simulink model "FIXEDPOINT_THIRD_ORDER_SIGMADELTA"  (R2021b)
settings: Solver=VariableStepAuto  StartTime=0.0  StopTime=0.1  MaxStep=1e-8  RelTol=1e-3
libraries: fl_lib x9, nesl_utility x4, simulink x1
settings Model: FPTShortcutValueString='{{},{''BaselineRun'',1,1,1,''BaselineRun'','''',{},''M'','''',''''},{''EmbeddedRun'',1,1,1,''EmbeddedRun'','''',{},''M'','''',''''}}'  Creator=caccolillo  LastModifiedBy=caccolillo
settings OptimizationCC: BlockReduction=off  ConditionallyExecuteInputs=off
settings DebuggingCC: SignalRangeChecking=warning

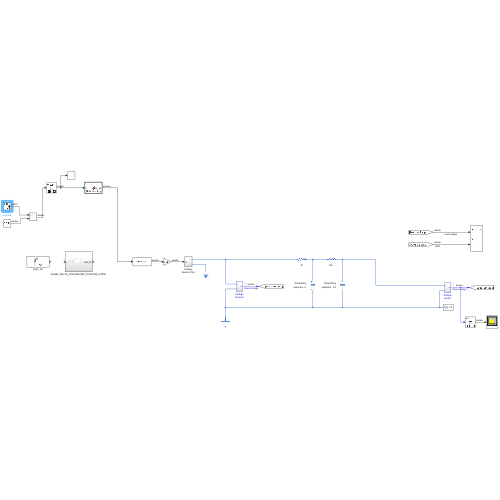
[thumbnail: Simulink's stored preview of the top-level diagram]
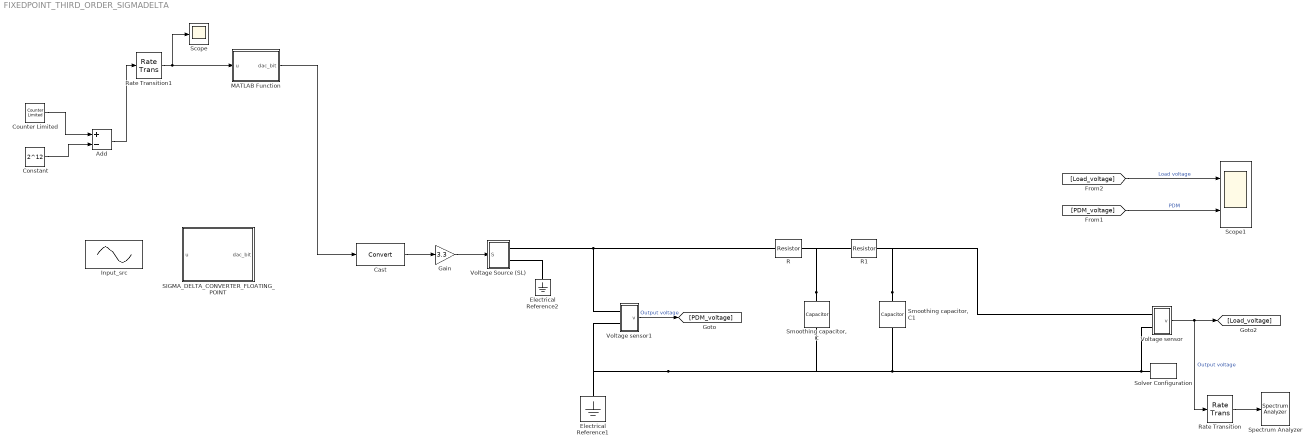
== system FIXEDPOINT_THIRD_ORDER_SIGMADELTA ==
  Add : Sum  Inputs=+-
  Cast : DataTypeConversion
  Constant : Constant  Value=2^12
  Counter Limited : simulink/Sources/Counter Limited  uplimit=2^13  tsamp=1/32000
  Electrical Reference1 : fl_lib/Electrical/Electrical Elements/Electrical Reference
  Electrical Reference2 : fl_lib/Electrical/Electrical Elements/Electrical Reference
  Gain : Gain  Gain=3.3
  Input_src : Sin  Amplitude=1024  Frequency=2*pi*1000  SampleTime=2e-07
  MATLAB Function : MATLAB Function  TreatAsAtomicUnit=on
  R : fl_lib/Electrical/Electrical Elements/Resistor  R=1 kOhm  i_specify=off  i_priority=High  i=0 A  i_nominal_specify=off  i_nominal_unit=A  i_nominal_value=1  v_specify=off  v_priority=High  v=0 V  v_nominal_specify=off  v_nominal_unit=V  v_nominal_value=1
  R1 : fl_lib/Electrical/Electrical Elements/Resistor  R=1 kOhm  i_specify=off  i_priority=High  i=0 A  i_nominal_specify=off  i_nominal_unit=A  i_nominal_value=1  v_specify=off  v_priority=High  v=0 V  v_nominal_specify=off  v_nominal_unit=V  v_nominal_value=1
  Rate Transition : RateTransition  Deterministic=off  OutPortSampleTime=1/100e3
  Rate Transition1 : RateTransition  Deterministic=off
  SIGMA_DELTA_CONVERTER_FLOATING_POINT : Subsystem
  Scope : Scope
  Scope1 : Scope  NumInputPorts=2
  "Smoothing capacitor, C" : fl_lib/Electrical/Electrical Elements/Capacitor  c=10 nF  r=0 Ohm  g=0 1/Ohm  i_specify=off  i_priority=High  i=0 A  i_nominal_specify=off  i_nominal_unit=A  i_nominal_value=1  v_specify=off  v_priority=High  v=0 V  v_nominal_specify=off  v_nominal_unit=V  v_nominal_value=1  vc_specify=on  vc_priority=High  vc=0 V  vc_nominal_specify=off  vc_nominal_unit=V  vc_nominal_value=1
  "Smoothing capacitor, C1" : fl_lib/Electrical/Electrical Elements/Capacitor  c=10 nF  r=0 Ohm  g=0 1/Ohm  i_specify=off  i_priority=High  i=0 A  i_nominal_specify=off  i_nominal_unit=A  i_nominal_value=1  v_specify=off  v_priority=High  v=0 V  v_nominal_specify=off  v_nominal_unit=V  v_nominal_value=1  vc_specify=on  vc_priority=High  vc=0 V  vc_nominal_specify=off  vc_nominal_unit=V  vc_nominal_value=1
  Solver Configuration : nesl_utility/Solver Configuration  PhysicalDomain=network_engine_domain  SubClassName=solver  LeftPortType=input  RightPortType=generic  Tones=[]  Harmonics=[]  SimulateNoise=off  Profile=off  UseLocalSampling=off  EnableSwitchedLinearOptims=on  FrequencyDomain=off  UseCCode=off  RelTol=0.001  AbsTol=1e-06  MinStep=1e-09  ToWorkspace=off  RevertToSquareIcSolve=off  NumHomotopyIterations=100  PhasorMode=off  PhasorModeNumHarmonics=1  DoDC=off  ResidualTolerance=1e-9  UseLocalSolver=off  LocalSolverChoice=NE_BACKWARD_EULER_ADVANCER  LocalSolverSampleTime=1e-7  DoFixedCost=off  MaxNonlinIter=12  MaxModeIter=2  ComputeImpulses=off  ImpulseIterations=2  LinearAlgebra=Sparse  EquationFormulation=NE_TIME_EF  DelaysMemoryBudget=1024  AutomaticFiltering=on  FilteringTimeConstant=0.001  PartitionStorageMethod=AS_NEEDED  PartitionMemoryBudget=1024  PartitionMethod=FAST
      settings: SourceProductBaseCode=PW,SS
  Spectrum Analyzer : SpectrumAnalyzer
  Voltage Source (SL) : Subsystem
      settings: CopyFcn=set_param(gcb,'LinkStatus','none')
  Voltage sensor : Subsystem
      settings: CopyFcn=set_param(gcb,'LinkStatus','none')
  Voltage sensor1 : Subsystem
      settings: CopyFcn=set_param(gcb,'LinkStatus','none')
  wires:
  [PDM_voltage] -> Scope1/2  "PDM"
  Rate Transition/1 -> Spectrum Analyzer/1
  Voltage sensor/1(v) -> Rate Transition/1, [Load_voltage]  "Output voltage"
  Voltage sensor1/1(v) -> [PDM_voltage]  "Output voltage"
  Gain/1 -> Voltage Source (SL)/1(S)
  [Load_voltage] -> Scope1/1  "Load voltage"
  Cast/1 -> Gain/1
  Add/1 -> Rate Transition1/1
  MATLAB Function/1(dac_bit) -> Cast/1
  Counter Limited/1 -> Add/1
  Constant/1 -> Add/2
  Rate Transition1/1 -> Scope/1, MATLAB Function/1(u)
  connections:
  Solver Configuration/RConn1 -- Voltage sensor1/LConn2 -- Electrical Reference1/LConn1 -- "Smoothing capacitor, C"/RConn1 -- "Smoothing capacitor, C1"/RConn1 -- Voltage sensor/LConn2
  "Smoothing capacitor, C"/LConn1 -- R/LConn1 -- R1/RConn1
  "Smoothing capacitor, C1"/LConn1 -- R1/LConn1 -- Voltage sensor/LConn1
  Voltage sensor1/LConn1 -- R/RConn1 -- Voltage Source (SL)/RConn1
  Voltage Source (SL)/RConn2 -- Electrical Reference2/LConn1

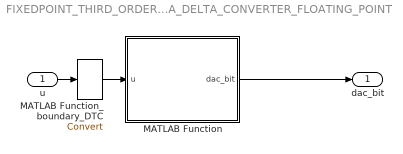
== system FIXEDPOINT_THIRD_ORDER_SIGMADELTA/SIGMA_DELTA_CONVERTER_FLOATING_POINT ==
  u : Inport
  MATLAB Function : Subsystem  TreatAsAtomicUnit=on  Variant=on  VariantControlMode=label  VariantControl=Choice  LabelModeActiveChoice=(default)
  MATLAB Function_boundary_DTC : DataTypeConversion  SaturateOnIntegerOverflow=on  RndMeth=Zero
  dac_bit : Outport
  wires:
  u/1 -> MATLAB Function_boundary_DTC/1
  MATLAB Function_boundary_DTC/1 -> MATLAB Function/1(u)
  MATLAB Function/1(dac_bit) -> dac_bit/1

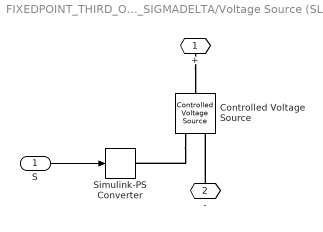
== system FIXEDPOINT_THIRD_ORDER_SIGMADELTA/Voltage Source (SL) ==
  S : Inport
  Controlled Voltage Source : fl_lib/Electrical/Electrical Sources/Controlled Voltage Source
  Simulink-PS Converter : nesl_utility/Simulink-PS Converter  PhysicalDomain=network_engine_domain  SubClassName=ps_input  LeftPortType=input  RightPortType=output  PseudoPeriodic=off  Frequencies=[]  NoiseDistribution=none  NoiseParameters=[]  Unit=V  AffineConversion=off  FilteringAndDerivatives=zero  SimscapeFilterOrder=1  InputFilterTimeConstant=.001  UdotUserProvided=0
      settings: SourceProductBaseCode=PW,SS
  + : PMIOPort  Side=Right
  - : PMIOPort  Port=2  Side=Right
  wires:
  S/1 -> Simulink-PS Converter/1
  connections:
  +/RConn1 -- Controlled Voltage Source/LConn1
  -/RConn1 -- Controlled Voltage Source/RConn2
  Controlled Voltage Source/RConn1 -- Simulink-PS Converter/RConn1

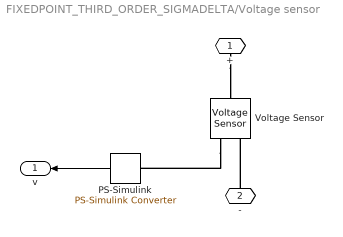
== system FIXEDPOINT_THIRD_ORDER_SIGMADELTA/Voltage sensor ==
  PS-Simulink : nesl_utility/PS-Simulink Converter  PhysicalDomain=network_engine_domain  SubClassName=ps_output  LeftPortType=input  RightPortType=output  PseudoPeriodic=off  Frequencies=[]  Unit=V  AffineConversion=off
      settings: SourceProductBaseCode=PW,SS
  Voltage Sensor : fl_lib/Electrical/Electrical Sensors/Voltage Sensor
  + : PMIOPort  Side=Left
  - : PMIOPort  Port=2  Side=Left
  v : Outport
  wires:
  PS-Simulink/1 -> v/1
  connections:
  Voltage Sensor/RConn1 -- PS-Simulink/LConn1
  +/RConn1 -- Voltage Sensor/LConn1
  -/RConn1 -- Voltage Sensor/RConn2

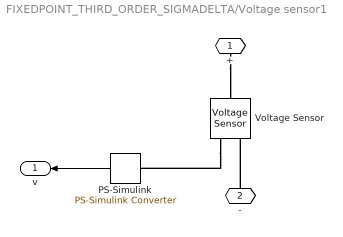
== system FIXEDPOINT_THIRD_ORDER_SIGMADELTA/Voltage sensor1 ==
  PS-Simulink : nesl_utility/PS-Simulink Converter  PhysicalDomain=network_engine_domain  SubClassName=ps_output  LeftPortType=input  RightPortType=output  PseudoPeriodic=off  Frequencies=[]  Unit=V  AffineConversion=off
      settings: SourceProductBaseCode=PW,SS
  Voltage Sensor : fl_lib/Electrical/Electrical Sensors/Voltage Sensor
  + : PMIOPort  Side=Left
  - : PMIOPort  Port=2  Side=Left
  v : Outport
  wires:
  PS-Simulink/1 -> v/1
  connections:
  Voltage Sensor/RConn1 -- PS-Simulink/LConn1
  +/RConn1 -- Voltage Sensor/LConn1
  -/RConn1 -- Voltage Sensor/RConn2

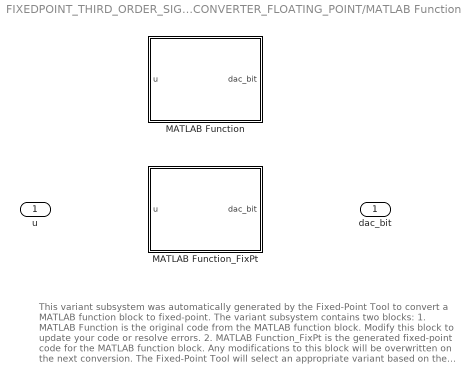
== system FIXEDPOINT_THIRD_ORDER_SIGMADELTA/SIGMA_DELTA_CONVERTER_FLOATING_POINT/MATLAB Function ==
  note: This variant subsystem was automatically generated by the Fixed-Point Tool to convert a MATLAB function block to fixed-point.
      |
      | The variant subsystem contains two blocks:
      | 1. MATLAB Function is the original code from the MATLAB function block. Modify this block to update your code or resolve errors.
      |
      | 2. MATLAB Function_FixPt is the generated fixed-point code for the MATLAB function block. Any modifications to this block will be overwritten on the next conversion.
      |
      | The Fixed-Point Tool will select an appropriate variant based on the Model Settings. Learn more. .
  u : Inport
  MATLAB Function : MATLAB Function  TreatAsAtomicUnit=on  VariantControl=false()
  MATLAB Function_FixPt : MATLAB Function  TreatAsAtomicUnit=on  VariantControl=(default)
  dac_bit : Outport

== matlab function FIXEDPOINT_THIRD_ORDER_SIGMADELTA/SIGMA_DELTA_CONVERTER_FLOATING_POINT/MATLAB Function/MATLAB Function_FixPt ==
  settings: fimath=fimath('RoundingMethod', 'Floor', 'OverflowAction', 'Wrap', 'ProductMode', 'FullPrecision', 'MaxProductWordLength', 128, 'SumMode', 'FullPrecision', 'MaxSumWordLength', 128)
  data: u input; dac_bit output
%auto-generated
function dac_bit = SDM_fcn_fixpt(u)  %#codegen
% Auto-generated by DESIGN_THIRD_ORDER.m
% 3rd-order CIFB sigma-delta modulator - FLOATING POINT REFERENCE
%
% This file is the floating-point golden model intended for use with
% MATLAB Fixed-Point Designer ("Convert to Fixed Point" workflow).
% All arithmetic uses double precision so the tool can instrument the
% function, observe min/max ranges, and propose data types.
%
% Input  u : signed integer count from the 13-bit ADC,
%            range [-4096, 4095]. Internally normalised to [-1,+1).
% Output : single bit (logical) for 1-bit DAC drive.
%
% Suggested starting types for Fixed-Point Designer:
%   u           : fixdt(1, 13, 0)
%   coefficients: fixdt(1, 18, 14)
%   int1..int3  : fixdt(1, 32, 14)

fm = get_fimath();
u = fi(u, 1, 16, 4, fm);

dac_bit = false;

persistent int1 int2 int3
if isempty(int1)
    int1 = fi(0, 1, 16, 15, fm);
    int2 = fi(0, 1, 16, 16, fm);
    int3 = fi(0, 1, 16, 17, fm);
end

% Floating-point coefficients (scaled CIFB, 3rd order)
B1 = fi(0.172222623529955, 0, 16, 18, fm);
A1 = fi(0.172222623529955, 0, 16, 18, fm);
A2 = fi(0.123562088507108, 0, 16, 18, fm);
A3 = fi(0.122457379474687, 0, 16, 19, fm);
C1 = fi(0.10952288682635, 0, 16, 19, fm);
C2 = fi(0.357050181625205, 0, 16, 17, fm);
G1 = fi(4.2457997600222e-05, 0, 16, 30, fm);

% Saturate and normalise the 13-bit signed input to [-1, +1)
u_sat = fi(max(min(double(u), fi(4095, 0, 12, 0, fm)), fi(-4096, 1, 13, 0, fm)), 1, 16, 4, fm);
u_norm = fi(fi_div_by_shift(u_sat, 12), 1, 16, 16, fm);

% Quantizer decision based on the last integrator (int3)
if int3 >= fi(0, 0, 1, 0, fm)
    dac_bit(:) = true;
    v       =  fi(1, 1, 16, 14, fm);
else
    dac_bit(:) = false;
    v       = fi(-1, 1, 16, 14, fm);
end

% Integrator 1: int1 += B1*u - A1*v
int1(:) = fi_signed(int1 + B1*u_norm) - A1*v;

% Integrator 2: int2 += C1*int1 - A2*v
int2(:) = fi_signed(int2 + C1*int1) - A2*v;

% Integrator 3: int3 += C2*int2 - G1*int3 - A3*v
% G1 is the resonator local feedback that places NTF zeros
% at non-DC frequencies inside the signal band.
int3(:) = fi_signed(fi_signed(int3 + C2*int2) - G1*int3) - A3*v;

end



function y = fi_div_by_shift(a,shift_len)
    coder.inline( 'always' );
    if isfi( a )
        nt = numerictype( a );
        fm = fimath( a );
        nt_bs = numerictype( nt.Signed, nt.WordLength + shift_len, nt.FractionLength + shift_len );
        y = bitsra( fi( a, nt_bs, fm ), shift_len );
    else
        y = a / 2 ^ shift_len;
    end
end


function y = fi_signed(a)
    coder.inline( 'always' );
    if isfi( a ) && ~(issigned( a ))
        nt = numerictype( a );
        new_nt = numerictype( 1, nt.WordLength + 1, nt.FractionLength );
        y = fi( a, new_nt, fimath( a ) );
    else
        y = a;
    end
end

function fm = get_fimath()
	fm = fimath('RoundingMethod', 'Floor',...
	     'OverflowAction', 'Wrap',...
	     'ProductMode','FullPrecision',...
	     'MaxProductWordLength', 128,...
	     'SumMode','FullPrecision',...
	     'MaxSumWordLength', 128);
end

== matlab function FIXEDPOINT_THIRD_ORDER_SIGMADELTA/MATLAB Function ==
  data: u input; dac_bit output
%auto-generated
function dac_bit = SDM_fcn_fixpt(u)  %#codegen
% Auto-generated by DESIGN_THIRD_ORDER.m
% 3rd-order CIFB sigma-delta modulator - FLOATING POINT REFERENCE
%
% This file is the floating-point golden model intended for use with
% MATLAB Fixed-Point Designer ("Convert to Fixed Point" workflow).
% All arithmetic uses double precision so the tool can instrument the
% function, observe min/max ranges, and propose data types.
%
% Input  u : signed integer count from the 13-bit ADC,
%            range [-4096, 4095]. Internally normalised to [-1,+1).
% Output : single bit (logical) for 1-bit DAC drive.
%
% Suggested starting types for Fixed-Point Designer:
%   u           : fixdt(1, 13, 0)
%   coefficients: fixdt(1, 18, 14)
%   int1..int3  : fixdt(1, 32, 14)

fm = get_fimath();
u = fi(u, 1, 16, 4, fm);

dac_bit = false;

persistent int1 int2 int3
if isempty(int1)
    int1 = fi(0, 1, 16, 15, fm);
    int2 = fi(0, 1, 16, 16, fm);
    int3 = fi(0, 1, 16, 17, fm);
end

% Floating-point coefficients (scaled CIFB, 3rd order)
B1 = fi(0.172222623529955, 0, 16, 18, fm);
A1 = fi(0.172222623529955, 0, 16, 18, fm);
A2 = fi(0.123562088507108, 0, 16, 18, fm);
A3 = fi(0.122457379474687, 0, 16, 19, fm);
C1 = fi(0.10952288682635, 0, 16, 19, fm);
C2 = fi(0.357050181625205, 0, 16, 17, fm);
G1 = fi(4.2457997600222e-05, 0, 16, 30, fm);

% Saturate and normalise the 13-bit signed input to [-1, +1)
u_sat = fi(max(min(double(u), fi(4095, 0, 12, 0, fm)), fi(-4096, 1, 13, 0, fm)), 1, 16, 4, fm);
u_norm = fi(fi_div_by_shift(u_sat, 12), 1, 16, 16, fm);

% Quantizer decision based on the last integrator (int3)
if int3 >= fi(0, 0, 1, 0, fm)
    dac_bit(:) = true;
    v       =  fi(1, 1, 16, 14, fm);
else
    dac_bit(:) = false;
    v       = fi(-1, 1, 16, 14, fm);
end

% Integrator 1: int1 += B1*u - A1*v
int1(:) = fi_signed(int1 + B1*u_norm) - A1*v;

% Integrator 2: int2 += C1*int1 - A2*v
int2(:) = fi_signed(int2 + C1*int1) - A2*v;

% Integrator 3: int3 += C2*int2 - G1*int3 - A3*v
% G1 is the resonator local feedback that places NTF zeros
% at non-DC frequencies inside the signal band.
int3(:) = fi_signed(fi_signed(int3 + C2*int2) - G1*int3) - A3*v;

end



function y = fi_div_by_shift(a,shift_len)
    coder.inline( 'always' );
    if isfi( a )
        nt = numerictype( a );
        fm = fimath( a );
        nt_bs = numerictype( nt.Signed, nt.WordLength + shift_len, nt.FractionLength + shift_len );
        y = bitsra( fi( a, nt_bs, fm ), shift_len );
    else
        y = a / 2 ^ shift_len;
    end
end


function y = fi_signed(a)
    coder.inline( 'always' );
    if isfi( a ) && ~(issigned( a ))
        nt = numerictype( a );
        new_nt = numerictype( 1, nt.WordLength + 1, nt.FractionLength );
        y = fi( a, new_nt, fimath( a ) );
    else
        y = a;
    end
end

function fm = get_fimath()
	fm = fimath('RoundingMethod', 'Floor',...
	     'OverflowAction', 'Wrap',...
	     'ProductMode','FullPrecision',...
	     'MaxProductWordLength', 128,...
	     'SumMode','FullPrecision',...
	     'MaxSumWordLength', 128);
end

== matlab function FIXEDPOINT_THIRD_ORDER_SIGMADELTA/SIGMA_DELTA_CONVERTER_FLOATING_POINT/MATLAB Function/MATLAB Function ==
  data: u input; dac_bit output
function dac_bit = SDM_fcn(u)  %#codegen
% Auto-generated by DESIGN_THIRD_ORDER.m
% 3rd-order CIFB sigma-delta modulator - FLOATING POINT REFERENCE
%
% This file is the floating-point golden model intended for use with
% MATLAB Fixed-Point Designer ("Convert to Fixed Point" workflow).
% All arithmetic uses double precision so the tool can instrument the
% function, observe min/max ranges, and propose data types.
%
% Input  u : signed integer count from the 13-bit ADC,
%            range [-4096, 4095]. Internally normalised to [-1,+1).
% Output : single bit (logical) for 1-bit DAC drive.
%
% Suggested starting types for Fixed-Point Designer:
%   u           : fixdt(1, 13, 0)
%   coefficients: fixdt(1, 18, 14)
%   int1..int3  : fixdt(1, 32, 14)

dac_bit = false;

persistent int1 int2 int3
if isempty(int1)
    int1 = 0;
    int2 = 0;
    int3 = 0;
end

% Floating-point coefficients (scaled CIFB, 3rd order)
B1 = 0.172222623529955;
A1 = 0.172222623529955;
A2 = 0.123562088507108;
A3 = 0.122457379474687;
C1 = 0.10952288682635;
C2 = 0.357050181625205;
G1 = 4.2457997600222e-05;

% Saturate and normalise the 13-bit signed input to [-1, +1)
u_sat = max(min(double(u), 4095), -4096);
u_norm = u_sat / 4096;

% Quantizer decision based on the last integrator (int3)
if int3 >= 0
    dac_bit = true;
    v       =  1;
else
    dac_bit = false;
    v       = -1;
end

% Integrator 1: int1 += B1*u - A1*v
int1 = int1 + B1*u_norm - A1*v;

% Integrator 2: int2 += C1*int1 - A2*v
int2 = int2 + C1*int1 - A2*v;

% Integrator 3: int3 += C2*int2 - G1*int3 - A3*v
% G1 is the resonator local feedback that places NTF zeros
% at non-DC frequencies inside the signal band.
int3 = int3 + C2*int2 - G1*int3 - A3*v;

end
